simulink model "lim_s_function"  (R2018a)
settings: Solver=ode4  StartTime=0.0  StopTime=100*pi  FixedStep=1e-5  MaxStep=1  RelTol=1e-3
libraries: simulink x1, powerlib_meascontrol x1
settings Model: Creator=QAQ  LastModifiedBy=akashsin
settings CodeAppCC: StateflowObjectComments=on

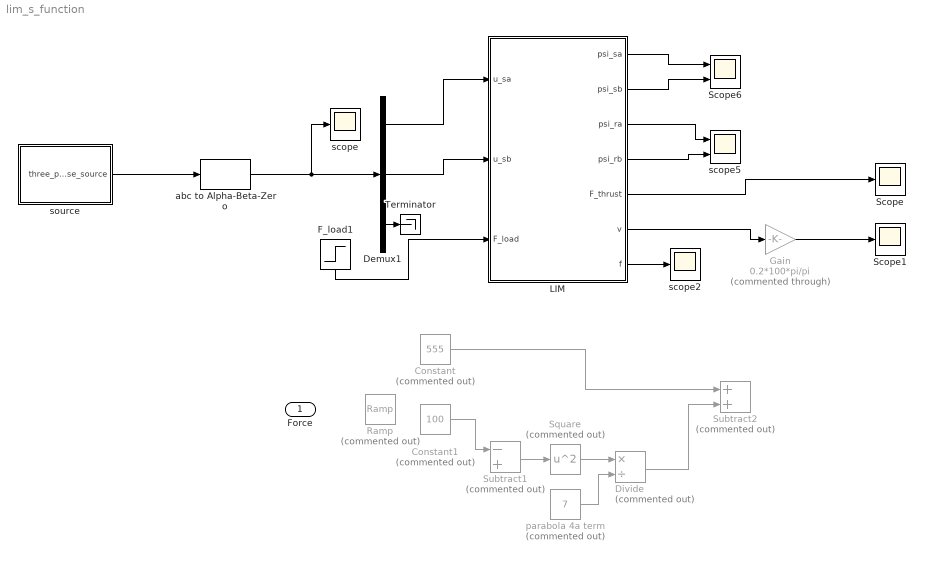
== system lim_s_function ==
  Force : Inport
  Constant : Constant  Commented=on  Value=555
  Constant1 : Constant  Commented=on  Value=100
  Demux1 : Demux  Outputs=3
  Divide : Product  Commented=on  Inputs=*/
  F_load1 : Step  Time=5e-2  After=0  SampleTime=5e-4
  Gain : Gain  Commented=through  Gain=0.2*100*pi/pi
  LIM : Subsystem
  Ramp : simulink/Sources/Ramp  Commented=on  slope=1000  start=10  InitialOutput=0  VectorParams1D=off
  Scope : Scope
  Scope1 : Scope
  Scope6 : Scope  NumInputPorts=2
  Square : Math  Commented=on  Operator=square  SaturateOnIntegerOverflow=on
  Subtract1 : Sum  Commented=on  Inputs=-+
  Subtract2 : Sum  Commented=on
  Terminator : Terminator
  abc to Alpha-Beta-Zero : powerlib_meascontrol/Transformations/abc to Alpha-Beta-Zero
      settings: SourceProductName=Simscape Power Systems
  parabola 4a term : Constant  Commented=on  Value=7
  scope : Scope
  scope2 : Scope
  scope5 : Scope  NumInputPorts=2
  source : Subsystem
  wires:
  Demux1/1 -> LIM/1(u_sa)
  Demux1/2 -> LIM/2(u_sb)
  LIM/2(psi_sb) -> Scope6/2
  LIM/1(psi_sa) -> Scope6/1
  LIM/3(psi_ra) -> scope5/1
  LIM/4(psi_rb) -> scope5/2
  LIM/5(F_thrust) -> Scope/1
  LIM/6(v) -> Gain/1
  Subtract1/1 -> Square/1
  Divide/1 -> Subtract2/2
  parabola 4a term/1 -> Divide/2
  Constant/1 -> Subtract2/1
  Constant1/1 -> Subtract1/1
  Square/1 -> Divide/1
  LIM/7(f) -> scope2/1
  F_load1/1 -> LIM/3(F_load)
  source/1(three_phase_source) -> abc to Alpha-Beta-Zero/1
  abc to Alpha-Beta-Zero/1 -> scope/1, Demux1/1
  Demux1/3 -> Terminator/1
  Gain/1 -> Scope1/1

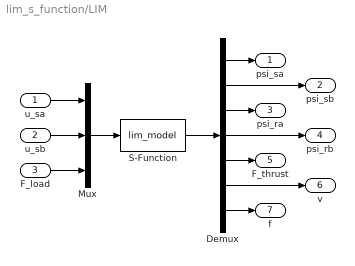
== system lim_s_function/LIM ==
  u_sa : Inport
  u_sb : Inport  Port=2
  F_load : Inport  Port=3
  Demux : Demux  Outputs=7
  Mux : Mux  Inputs=3
  S-Function : S-Function  FunctionName=lim_model  SFunctionDeploymentMode=off  EnableBusSupport=off
  psi_sa : Outport
  psi_sb : Outport  Port=2
  psi_ra : Outport  Port=3
  psi_rb : Outport  Port=4
  F_thrust : Outport  Port=5
  v : Outport  Port=6
  f : Outport  Port=7
  wires:
  Mux/1 -> S-Function/1
  u_sa/1 -> Mux/1
  u_sb/1 -> Mux/2
  F_load/1 -> Mux/3
  S-Function/1 -> Demux/1
  Demux/2 -> psi_sb/1
  Demux/1 -> psi_sa/1
  Demux/3 -> psi_ra/1
  Demux/5 -> F_thrust/1
  Demux/4 -> psi_rb/1
  Demux/6 -> v/1
  Demux/7 -> f/1

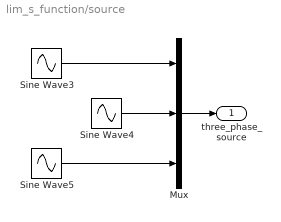
== system lim_s_function/source ==
  Mux : Mux  Inputs=3
  Sine Wave3 : Sin  SampleTime=0
  Sine Wave4 : Sin  Phase=-2*pi/3  SampleTime=0
  Sine Wave5 : Sin  Phase=2*pi/3  SampleTime=0
  three_phase_source : Outport
  wires:
  Sine Wave5/1 -> Mux/3
  Sine Wave3/1 -> Mux/1
  Mux/1 -> three_phase_source/1
  Sine Wave4/1 -> Mux/2
